simulink model "simulation"  (R2014b)
settings: Solver=ode45  StartTime=0.0  StopTime=500.0  FixedStep=n  MaxStep=n  MinStep=0.0001  RelTol=1e-3
values from neighbouring files (symbols this model uses):
  k = 3.1    [dane.m]    (also in dane1.m)
  n = 10    [dane.m]    (also in dane1.m)
settings Model: Creator=podstawy  LastModifiedBy=podstawy

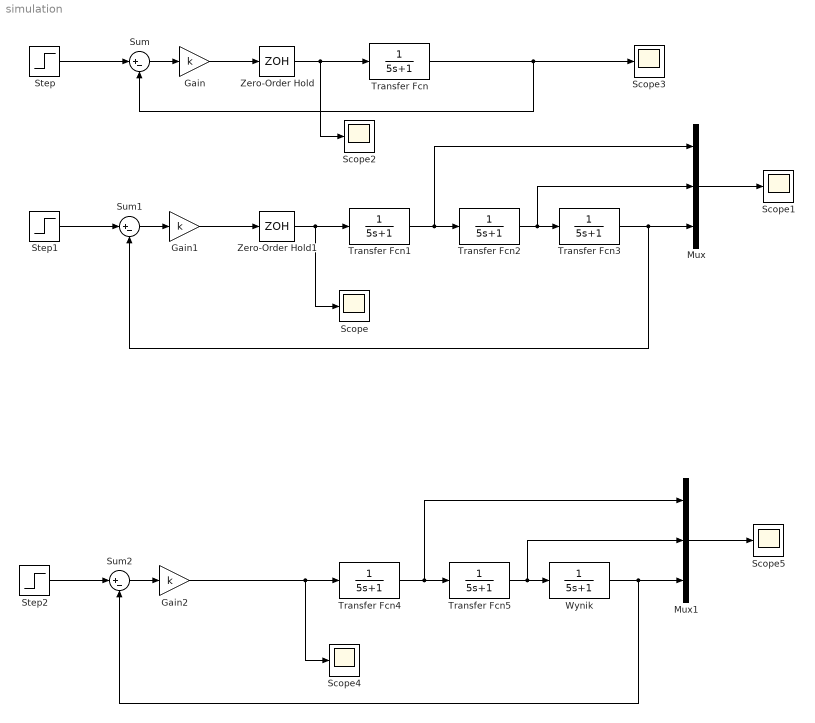
== system simulation ==
  Gain : Gain  Gain=k
  Gain1 : Gain  Gain=k
  Gain2 : Gain  Gain=k
  Mux : Mux  Inputs=3
  Mux1 : Mux  Inputs=3
  Scope{,1..5} (6 alike) : Scope
      Scope settings: SaveName=Sterowanie2
      Scope1 settings: ShowLegends=on  SaveName=Wynik2
      Scope2 settings: SaveName=Sterowanie1
      Scope3 settings: SaveName=Wynik1
      Scope4 settings: SaveName=Sterowanie3
      Scope5 settings: ShowLegends=on  SaveName=Wynik3
  Step : Step  Time=0  SampleTime=0
  Step1 : Step  Time=0  SampleTime=0
  Step2 : Step  Time=0  SampleTime=0
  Sum : Sum  Inputs=|+-
  Sum1 : Sum  Inputs=|+-
  Sum2 : Sum  Inputs=|+-
  Transfer Fcn{,1..5} (6 alike) : TransferFcn  Denominator=[5 1]
  Wynik : TransferFcn  Denominator=[5 1]
  Zero-Order Hold : ZeroOrderHold  SampleTime=n
  Zero-Order Hold1 : ZeroOrderHold  SampleTime=n
  wires:
  Mux/1 -> Scope1/1
  Step/1 -> Sum/1
  Sum/1 -> Gain/1
  Gain/1 -> Zero-Order Hold/1
  Zero-Order Hold/1 -> Scope2/1, Transfer Fcn/1
  Transfer Fcn/1 -> Sum/2, Scope3/1
  Step1/1 -> Sum1/1
  Sum1/1 -> Gain1/1
  Gain1/1 -> Zero-Order Hold1/1
  Zero-Order Hold1/1 -> Scope/1, Transfer Fcn1/1
  Transfer Fcn1/1 -> Mux/1, Transfer Fcn2/1
  Transfer Fcn2/1 -> Mux/2, Transfer Fcn3/1
  Transfer Fcn3/1 -> Sum1/2, Mux/3
  Mux1/1 -> Scope5/1
  Step2/1 -> Sum2/1
  Sum2/1 -> Gain2/1
  Gain2/1 -> Scope4/1, Transfer Fcn4/1
  Transfer Fcn4/1 -> Mux1/1, Transfer Fcn5/1
  Transfer Fcn5/1 -> Mux1/2, Wynik/1
  Wynik/1 -> Sum2/2, Mux1/3
